simulink model "heaterLygeros"  (Simulink 8.3)
settings: Solver=ode45  StartTime=0.0  StopTime=0.25  RelTol=1e-3
settings Model: Creator=tjohnson  LastModifiedBy=tjohnson
settings DataIOCC: SignalLoggingSaveFormat=Dataset
settings DebuggingCC: UnderspecifiedInitializationDetection=Simplified  StateNameClashWarn=none
settings GRTTargetCC: CombineOutputUpdateFcns=on  GRTInterface=off

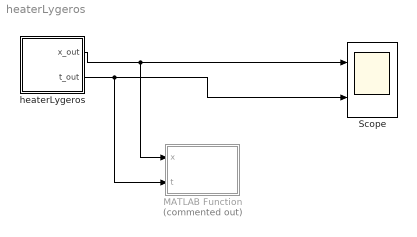
== system heaterLygeros ==
  MATLAB Function : MATLAB Function  Commented=on  TreatAsAtomicUnit=on
  Scope : Scope  NumInputPorts=2
      settings: YMin=-5~-5  YMax=5~5
  heaterLygeros : Stateflow chart  InitFcn='init'  StartFcn='start'  StopFcn='stop'  TreatAsAtomicUnit=on
      settings: PauseFcn='pause'  ContinueFcn='continue'
  wires:
  heaterLygeros/1(x_out) -> MATLAB Function/1(x), Scope/1
  heaterLygeros/2(t_out) -> MATLAB Function/2(t), Scope/2

== matlab function MATLAB Function ==
  data: x input double; t input double
function fcn(x,t)
%#codegen
coder.extrinsic('sprintf');

javaaddpath(['.', filesep, 'lib', filesep, 'daikon.jar']);
import  daikon.Runtime.dtrace.*;

    filesep = '/';
    opt_time = 1;
    
    simTime = t;
    simData = x;
    
    simTimeRep = strrep(sprintf('%.10f', simTime), '.', '_');
    
    %ppt_name = ['heaterLygeros:::POINT_t', simTimeRep];
    ppt_name = ['heaterLygeros:::POINT_t'];
    

    output_dir = ['daikon-output', filesep];
    output_filename = ['output_', simTimeRep, '.dtrace'];
    output_filepath = [output_dir, output_filename];

    %daikon.Runtime.no_dtrace = true;
    daikon.Runtime.setDtraceMaybe(output_filepath);
    daikon.Runtime.setDtrace(output_filepath, false); % todo: figure out which of these actually opens the file...

    daikon.Runtime.dtrace.println('input-language Simulink/Stateflow');
    daikon.Runtime.dtrace.println('decl-version 2.0');
    daikon.Runtime.dtrace.println('var-comparability implicit');
    daikon.Runtime.dtrace.println();


    
    daikon.Runtime.dtrace.println(['ppt ..', ppt_name]);
    daikon.Runtime.dtrace.println('  ppt-type point');
    if opt_time
        daikon.Runtime.dtrace.println('  variable ::time');
        daikon.Runtime.dtrace.println('    var-kind variable');
        daikon.Runtime.dtrace.println('    rep-type double');
        daikon.Runtime.dtrace.println('    dec-type double');
        daikon.Runtime.dtrace.println('    comparability 1');
    end
    daikon.Runtime.dtrace.println('  variable ::x');
    daikon.Runtime.dtrace.println('    var-kind variable');
    daikon.Runtime.dtrace.println('    rep-type double');
    daikon.Runtime.dtrace.println('    dec-type double');
    daikon.Runtime.dtrace.println('    comparability 2');
    
    
%     daikon.Runtime.dtrace.println('time:');
%     daikon.Runtime.dtrace.println(num2str(simTime));
%     daikon.Runtime.dtrace.println('variable:');
%     daikon.Runtime.dtrace.println(num2str(simData));
    daikon.Runtime.dtrace.println();
    daikon.Runtime.dtrace.println(['..', ppt_name]);
    if opt_time
        daikon.Runtime.dtrace.println('::time');
        daikon.Runtime.dtrace.println(num2str(simTime));
        daikon.Runtime.dtrace.println('1'); % always set as modified
    end
    daikon.Runtime.dtrace.println('::x');
    daikon.Runtime.dtrace.println(num2str(simData));
    daikon.Runtime.dtrace.println('1'); % always set as modified
    daikon.Runtime.dtrace.println();
    
    %daikon.Runtime.noMoreOutput(); % don't call this, will kill because it
    %sets no_dtrace to true
    daikon.Runtime.dtrace.close(); % flushes file
    %pause(0.01);

== stateflow chart heaterLygeros ==
  settings: updateMethod=CONTINUOUS
  state off
    du:
    x_dot=-8*x;
    t_dot=1;
    x_out=x;
    t_out=t;
  state on
    du:
    x_dot=-8*(x-30);
    t_dot=1;
    x_out=x;
    t_out=t;
  on -> off : [x>=22]
  (default) -> off : {x=18;t=0;}
  off -> on : [x<=18]
  data: x local double; x_out output double; t local double; t_out output double
  data x settings: updateMethod=SF_CONTINUOUS_TIME_DATA
  data t settings: updateMethod=SF_CONTINUOUS_TIME_DATA
